simulink model "RUNRUNRUN"  (Simulink 7.6)
settings: Solver=ode45  StartTime=0.0  StopTime=10.0  RelTol=1e-3
libraries: simulink x1
settings Model: Creator=TCA  LastModifiedBy=meuser
settings OptimizationCC: InitFltsAndDblsToZero=on
settings DebuggingCC: StrictBusMsg=Warning

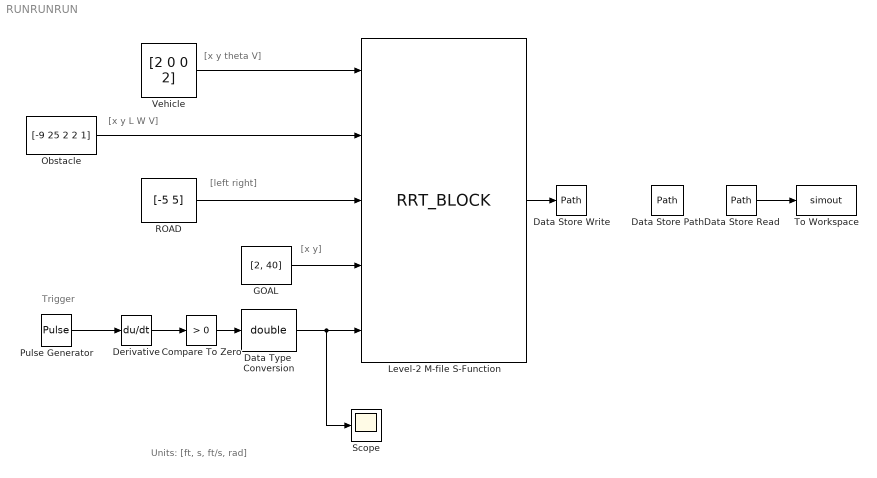
== system RUNRUNRUN ==
  note: [x y theta V]
  note: [x y L W V]
  note: [left right]
  note: [x y]
  note: Units: [ft, s, ft/s, rad]
  note: Trigger
  Compare To Zero : simulink/Logic and Bit Operations/Compare To Zero  SystemSampleTime=-1  relop=>  LogicOutDataTypeMode=uint8  ZeroCross=off
  Data Store Path : DataStoreMemory  DataStoreName=Path  ReadBeforeWriteMsg=warning  WriteAfterWriteMsg=warning  WriteAfterReadMsg=warning  InitialValue=zeros(50, 6)  VectorParams1D=off
  Data Store Read : DataStoreRead  DataStoreName=Path  SampleTime=0
  Data Store Write : DataStoreWrite  DataStoreName=Path
  Data Type  Conversion : DataTypeConversion  OutDataTypeStr=double  SaturateOnIntegerOverflow=on  RndMeth=Zero
  Derivative : Derivative
  GOAL : Constant  Value=[2, 40]  VectorParams1D=off
  Level-2 M-file S-Function : M-S-Function  FunctionName=RRT_BLOCK  Parameters=20
  Obstacle : Constant  Value=[-9 25 2 2 1]  VectorParams1D=off
  Pulse Generator : DiscretePulseGenerator  PulseType=Time based  Period=1  PulseWidth=5
  ROAD : Constant  Value=[-5 5]  VectorParams1D=off
  Scope : Scope
      settings: TimeRange=10  YMin=0  YMax=1
  To Workspace : ToWorkspace  VariableName=simout  SampleTime=-1  SaveFormat=Array
  Vehicle : Constant  Value=[2 0 0 2]  VectorParams1D=off
  wires:
  Vehicle/1 -> Level-2 M-file S-Function/1
  Obstacle/1 -> Level-2 M-file S-Function/2
  ROAD/1 -> Level-2 M-file S-Function/3
  GOAL/1 -> Level-2 M-file S-Function/4
  Data Store Read/1 -> To Workspace/1
  Compare To Zero/1 -> Data Type  Conversion/1
  Level-2 M-file S-Function/1 -> Data Store Write/1
  Pulse Generator/1 -> Derivative/1
  Data Type  Conversion/1 -> Level-2 M-file S-Function/5, Scope/1
  Derivative/1 -> Compare To Zero/1
